simulink library "Electric_Drive_Tabled_Consumption"  (R2018b)
settings: Solver=VariableStepAuto  StartTime=0.0  StopTime=10.0  RelTol=1e-3
undefined symbols (not defined in the file): OM_PEl_M_Map, PEl_MotVector
(part 2 of 2)

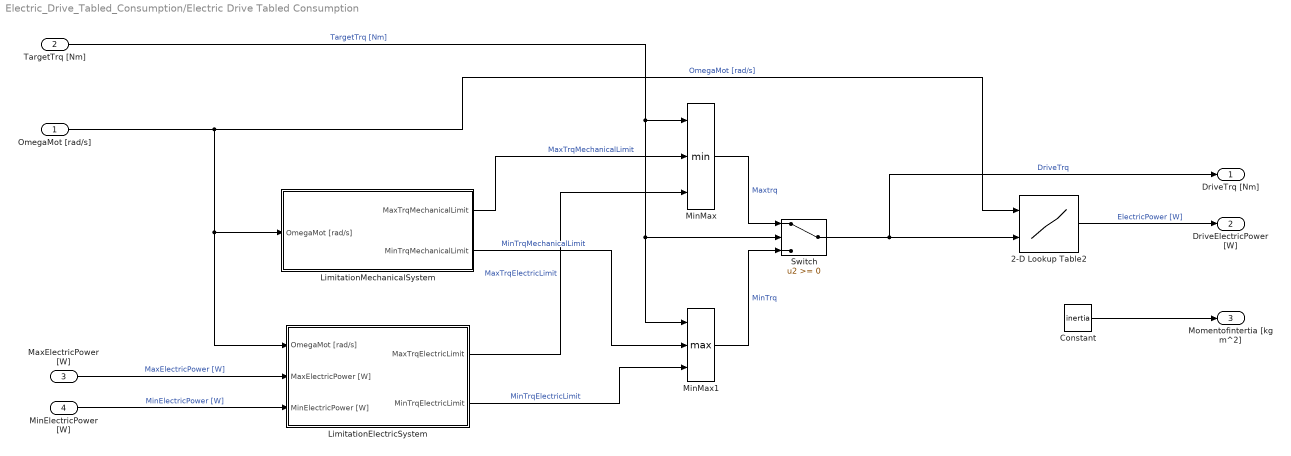
== system Electric_Drive_Tabled_Consumption/Electric Drive Tabled Consumption ==
  OmegaMot [rad/s] : Inport  SampleTime=LocalSampleTime
  TargetTrq [Nm] : Inport  Port=2  SampleTime=LocalSampleTime
  MaxElectricPower [W] : Inport  Port=3  SampleTime=LocalSampleTime
  MinElectricPower [W] : Inport  Port=4  SampleTime=LocalSampleTime
  2-D Lookup Table2 : Lookup_n-D  BreakpointsForDimension1=OM_MotVector  BreakpointsForDimension2=M_MotVector  Table=OM_M_Pel_Map  UseLastTableValue=on  InternalRulePriority=Speed  RndMeth=Simplest  InputSameDT=on
  Constant : Constant  Value=inertia
  LimitationElectricSystem : Subsystem
  LimitationMechanicalSystem : Subsystem
  MinMax : MinMax  Inputs=3
  MinMax1 : MinMax  Function=max  Inputs=3
  Switch : Switch
  DriveTrq [Nm] : Outport  SampleTime=GlobalSampleTime
  DriveElectricPower [W] : Outport  Port=2  SampleTime=GlobalSampleTime
  Momentofintertia [kg m^2] : Outport  Port=3  SampleTime=GlobalSampleTime
  wires:
  2-D Lookup Table2/1 -> DriveElectricPower [W]/1  "ElectricPower [W]"
  MinMax/1 -> Switch/1  "Maxtrq"
  MinMax1/1 -> Switch/3  "MinTrq"
  TargetTrq [Nm]/1 -> MinMax1/1, Switch/2, MinMax/1  "TargetTrq [Nm]"
  Switch/1 -> 2-D Lookup Table2/2, DriveTrq [Nm]/1  "DriveTrq"
  OmegaMot [rad/s]/1 -> LimitationElectricSystem/1(OmegaMot [rad/s]), LimitationMechanicalSystem/1(OmegaMot [rad/s]), 2-D Lookup Table2/1  "OmegaMot [rad/s]"
  MaxElectricPower [W]/1 -> LimitationElectricSystem/2(MaxElectricPower [W])  "MaxElectricPower [W]"
  MinElectricPower [W]/1 -> LimitationElectricSystem/3(MinElectricPower [W])  "MinElectricPower [W]"
  LimitationMechanicalSystem/1(MaxTrqMechanicalLimit) -> MinMax/2  "MaxTrqMechanicalLimit"
  LimitationMechanicalSystem/2(MinTrqMechanicalLimit) -> MinMax1/2  "MinTrqMechanicalLimit"
  LimitationElectricSystem/2(MinTrqElectricLimit) -> MinMax1/3  "MinTrqElectricLimit"
  LimitationElectricSystem/1(MaxTrqElectricLimit) -> MinMax/3  "MaxTrqElectricLimit"
  Constant/1 -> Momentofintertia [kg m^2]/1

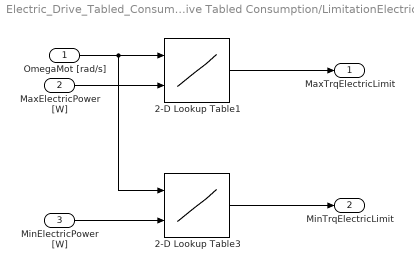
== system Electric_Drive_Tabled_Consumption/Electric Drive Tabled Consumption/LimitationElectricSystem ==
  OmegaMot [rad/s] : Inport
  MaxElectricPower [W] : Inport  Port=2
  MinElectricPower [W] : Inport  Port=3
  2-D Lookup Table1 : Lookup_n-D  BreakpointsForDimension1=OM_MotVector  BreakpointsForDimension2=PEl_MotVector  Table=OM_PEl_M_Map  UseLastTableValue=on  InternalRulePriority=Speed  RndMeth=Simplest  InputSameDT=on
  2-D Lookup Table3 : Lookup_n-D  BreakpointsForDimension1=OM_MotVector  BreakpointsForDimension2=PEl_MotVector  Table=OM_PEl_M_Map  UseLastTableValue=on  InternalRulePriority=Speed  RndMeth=Simplest  InputSameDT=on
  MaxTrqElectricLimit : Outport
  MinTrqElectricLimit : Outport  Port=2
  wires:
  MaxElectricPower [W]/1 -> 2-D Lookup Table1/2
  MinElectricPower [W]/1 -> 2-D Lookup Table3/2
  2-D Lookup Table3/1 -> MinTrqElectricLimit/1
  OmegaMot [rad/s]/1 -> 2-D Lookup Table3/1, 2-D Lookup Table1/1
  2-D Lookup Table1/1 -> MaxTrqElectricLimit/1

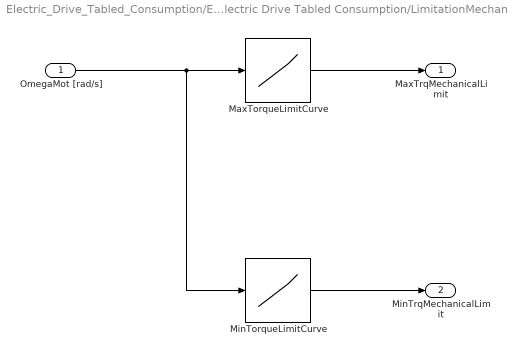
== system Electric_Drive_Tabled_Consumption/Electric Drive Tabled Consumption/LimitationMechanicalSystem ==
  OmegaMot [rad/s] : Inport
  MaxTorqueLimitCurve : Lookup_n-D  NumberOfTableDimensions=1  BreakpointsForDimension1=OM_Full_Load  Table=M_Full_Load  InternalRulePriority=Speed  RndMeth=Simplest  InputSameDT=on
  MinTorqueLimitCurve : Lookup_n-D  NumberOfTableDimensions=1  BreakpointsForDimension1=OM_Min_Load  Table=M_Min_Load  InternalRulePriority=Speed  RndMeth=Simplest  InputSameDT=on
  MaxTrqMechanicalLimit : Outport
  MinTrqMechanicalLimit : Outport  Port=2
  wires:
  MinTorqueLimitCurve/1 -> MinTrqMechanicalLimit/1
  MaxTorqueLimitCurve/1 -> MaxTrqMechanicalLimit/1
  OmegaMot [rad/s]/1 -> MaxTorqueLimitCurve/1, MinTorqueLimitCurve/1
